simulink model "Matlab_Model_Nagr_Butoma"  (R2018b)
settings: Solver=VariableStepAuto  StartTime=0.0  StopTime=0.2  RelTol=1e-3
libraries: powerlib x9, peRmsMeasurement x4
settings Model: Creator=sr1  LastModifiedBy=sr1

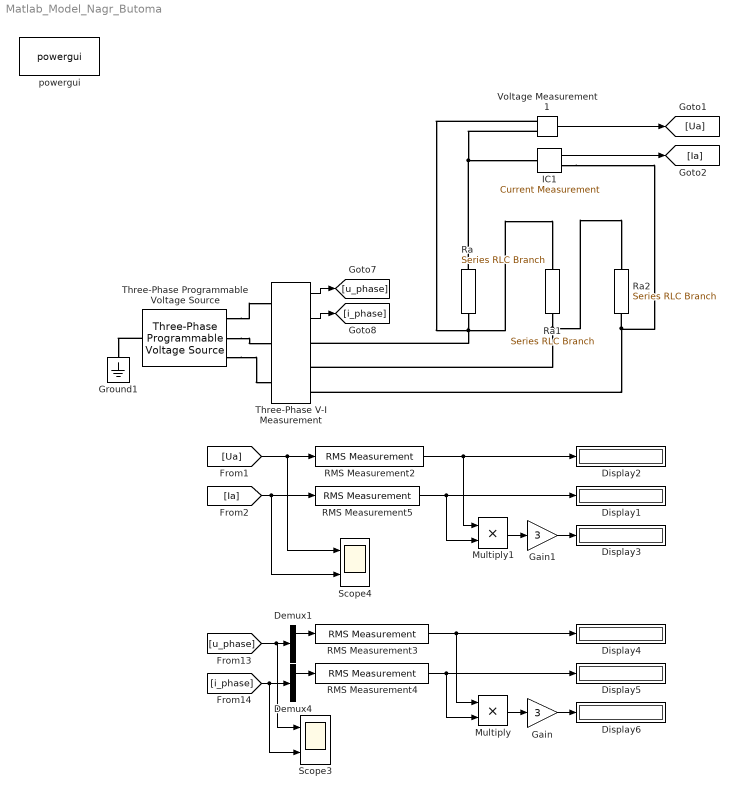
== system Matlab_Model_Nagr_Butoma ==
  Demux1 : Demux  Outputs=3
  Demux4 : Demux  Outputs=3
  Display{1..6} (6 alike) : Display
  Gain : Gain  Gain=3
  Gain1 : Gain  Gain=3
  Ground1 : powerlib/Elements/Ground  LConnTagsString=a
  IC1 : powerlib/Measurements/Current Measurement  PhasorSimulation=off  OutputType=Complex  PSBequivalent=0
  Multiply : Product
  Multiply1 : Product
  RMS Measurement{2..5} (4 alike) : peRmsMeasurement/RMS Measurement  LabelModeActiveChoice=Harmonic  F=50  SpecifyHarmonics=on  K=[1]  Ts=0
  Ra : powerlib/Elements/Series RLC Branch  LConnTagsString=__new0  RConnTagsString=__new0  BranchType=R  Resistance=16  Inductance=1e-3  SetiL0=off  InitialCurrent=0  Capacitance=1e-6  Setx0=off  InitialVoltage=0  Measurements=None
  Ra1 : powerlib/Elements/Series RLC Branch  LConnTagsString=__new0  RConnTagsString=__new0  BranchType=R  Resistance=16  Inductance=1e-3  SetiL0=off  InitialCurrent=0  Capacitance=1e-6  Setx0=off  InitialVoltage=0  Measurements=None
  Ra2 : powerlib/Elements/Series RLC Branch  LConnTagsString=__new0  RConnTagsString=__new0  BranchType=R  Resistance=16  Inductance=1e-3  SetiL0=off  InitialCurrent=0  Capacitance=1e-6  Setx0=off  InitialVoltage=0  Measurements=None
  Scope3 : Scope  NumInputPorts=2
  Scope4 : Scope  NumInputPorts=2
  Three-Phase Programmable Voltage Source : powerlib/Electrical Sources/Three-Phase Programmable Voltage Source  PositiveSequence=[208 0 50]  VariationEntity=None  VariationType=Table of time-amplitude pairs  VariationTypeAlt=Step  VariationStep=0.5  VariationRate=10  VariationMagnitude=0.3  VariationFrequency=2  VariationTiming=[1 2]  VariationPhaseA=off  Amplitudes=[1 0.8 1.2 1.0]  TimeValues=[0 0.1 0.15 0.2]  HarmonicGeneration=off  HarmonicA=[3 0.2 -25 0]  HarmonicB=[2 0.15 35 2]  Timing="[0.05  3]"  BusType=swing  Pref=0  Qref=0  Qmin=-inf  Qmax=inf
  Three-Phase V-I Measurement : powerlib/Measurements/Three-Phase V-I Measurement  VoltageMeasurement=phase-to-ground  SetLabelV=off  LabelV=Vabc  Vpu=off  VpuLL=off  CurrentMeasurement=yes  SetLabelI=off  LabelI=Iabc  Ipu=off  Pbase=100e6  Vbase=500e3  OutputType=Complex  PhasorSimulation=off  PSBequivalent=0
  Voltage Measurement1 : powerlib/Measurements/Voltage Measurement  PhasorSimulation=off  OutputType=Complex  PSBequivalent=0
  powergui : powerlib/powergui  Priority=1  SimulationMode=Discrete  SampleTime=1e-7  frequency=60  Iterations=50  frequencyindice=50  Pbase=100e6  ErrMax=1e-4  UnitsV=kV  UnitsW=MW  buscounter=0  FunctionMessages=off  echomessages=off  EnableUseOfTLC=off  CurrentSourceSwitches=off  DisableSnubberDevices=off  DisableRonSwitches=off  DisableVfSwitches=off  DisplayEquations=off  SolverType=Tustin/Backward Euler (TBE)  Interpol=off  ExternalGateDelay=off  methode=off  Ts=100  x0status=blocks  SPID=on  SwTol=0  HookPort=off  RestoreLinks=warning  ResistiveCurrentMeasurement=off  Frange=[0:2:500]  Ylog=off  Xlog=on  ShowGrid=off  save=off  variable=ZData  structure=0  ZoomFFT=off  StartTime=0.0  cycles=1  DisplayStyle=1  fundamental=60  FreqAxis=off  MaxFrequency=1000  frequencyindicesteady=1  RmsSteady=1  display=off
  wires:
  Three-Phase V-I Measurement/2 -> [i_phase]
  Three-Phase V-I Measurement/1 -> [u_phase]
  RMS Measurement4/1 -> Display5/1, Multiply/2
  [i_phase] -> Demux4/1, Scope3/2
  [u_phase] -> Scope3/1, Demux1/1
  Multiply/1 -> Gain/1
  Gain/1 -> Display6/1
  RMS Measurement3/1 -> Display4/1, Multiply/1
  Demux4/1 -> RMS Measurement4/1
  Demux1/1 -> RMS Measurement3/1
  Voltage Measurement1/1 -> [Ua]
  IC1/1 -> [Ia]
  [Ia] -> RMS Measurement5/1, Scope4/2
  Multiply1/1 -> Gain1/1
  Gain1/1 -> Display3/1
  RMS Measurement2/1 -> Multiply1/1, Display2/1
  RMS Measurement5/1 -> Display1/1, Multiply1/2
  [Ua] -> RMS Measurement2/1, Scope4/1
  connections:
  Three-Phase Programmable Voltage Source/RConn1 -- Three-Phase V-I Measurement/LConn1
  Three-Phase Programmable Voltage Source/LConn1 -- Ground1/LConn1
  Three-Phase Programmable Voltage Source/RConn3 -- Three-Phase V-I Measurement/LConn3
  Three-Phase Programmable Voltage Source/RConn2 -- Three-Phase V-I Measurement/LConn2
  Ra/RConn1 -- Three-Phase V-I Measurement/RConn1 -- Voltage Measurement1/LConn1 -- Ra1/LConn1
  Ra1/RConn1 -- Three-Phase V-I Measurement/RConn2 -- Ra2/LConn1
  Ra2/RConn1 -- Three-Phase V-I Measurement/RConn3 -- IC1/RConn1
  Ra/LConn1 -- IC1/LConn1 -- Voltage Measurement1/LConn2
